simulink model "Question2f"  (R2018a)
settings: Solver=VariableStepAuto  StartTime=0.0  StopTime=15  RelTol=1e-3
settings Model: Creator=e217715  LastModifiedBy=e227863

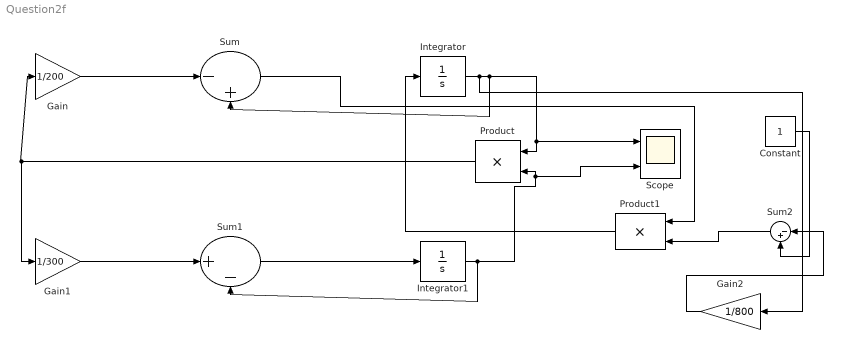
== system Question2f ==
  Constant : Constant
  Gain : Gain  Gain=1/200
  Gain1 : Gain  Gain=1/300
  Gain2 : Gain  Gain=1/800
  Integrator : Integrator  InitialCondition=400
  Integrator1 : Integrator  InitialCondition=100
  Product : Product
  Product1 : Product
  Scope : Scope  NumInputPorts=2
  Sum : Sum  Inputs=|-+
  Sum1 : Sum  Inputs=|+-
  Sum2 : Sum  Inputs=|-+
  wires:
  Gain/1 -> Sum/1
  Gain1/1 -> Sum1/1
  Sum1/1 -> Integrator1/1
  Integrator/1 -> Gain2/1, Sum/2, Product/1, Scope/1
  Integrator1/1 -> Sum1/2, Scope/2, Product/2
  Product/1 -> Gain1/1, Gain/1
  Sum/1 -> Product1/1
  Sum2/1 -> Product1/2
  Product1/1 -> Integrator/1
  Constant/1 -> Sum2/2
  Gain2/1 -> Sum2/1
